simulink model "ground_state_nonridgid"  (R2017b)
settings: Solver=VariableStepAuto  StartTime=0.0  StopTime=10  RelTol=1e-3
undefined symbols (not defined in the file or in its folder): refo
settings Model: Creator=benma  LastModifiedBy=benma

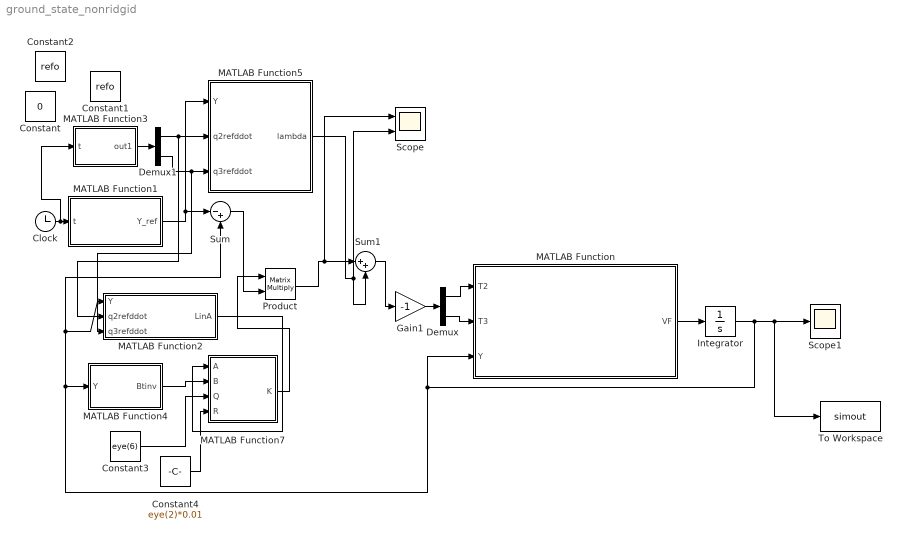
== system ground_state_nonridgid ==
  Clock : Clock
  Constant : Constant  Value=0
  Constant1 : Constant  Value=refo
  Constant2 : Constant  Value=refo
  Constant3 : Constant  Value=eye(6)
  Constant4 : Constant  Value=eye(2)*0.01
  Demux : Demux  Outputs=2
  Demux1 : Demux  Outputs=2
  Gain1 : Gain  Gain=-1
  Integrator : Integrator  InitialCondition=refo
  MATLAB Function : MATLAB Function  TreatAsAtomicUnit=on
  MATLAB Function1 : MATLAB Function  TreatAsAtomicUnit=on
  MATLAB Function2 : MATLAB Function  TreatAsAtomicUnit=on
  MATLAB Function3 : MATLAB Function  TreatAsAtomicUnit=on
  MATLAB Function4 : MATLAB Function  TreatAsAtomicUnit=on
  MATLAB Function5 : MATLAB Function  TreatAsAtomicUnit=on
  MATLAB Function7 : MATLAB Function  TreatAsAtomicUnit=on
  Product : Product  Multiplication=Matrix(*)
  Scope : Scope  NumInputPorts=2
  Scope1 : Scope
  Sum : Sum  Inputs=|-+
  Sum1 : Sum  Inputs=|++
  To Workspace : ToWorkspace  VariableName=simout  SaveFormat=Timeseries  SampleTime=-1
  wires:
  MATLAB Function/1(VF) -> Integrator/1
  Gain1/1 -> Demux/1
  Demux/1 -> MATLAB Function/1(T2)
  Demux/2 -> MATLAB Function/2(T3)
  MATLAB Function5/1(lambda) -> Sum1/2, Scope/2
  Sum1/1 -> Gain1/1
  Clock/1 -> MATLAB Function3/1(t), MATLAB Function1/1(t)
  MATLAB Function1/1(Y_ref) -> Sum/1, MATLAB Function5/1(Y)
  Integrator/1 -> To Workspace/1, Scope1/1, MATLAB Function/3(Y), MATLAB Function4/1(Y), MATLAB Function2/1(Y), Sum/2
  MATLAB Function2/1(LinA) -> MATLAB Function7/1(A)
  MATLAB Function4/1(Btinv) -> MATLAB Function7/2(B)
  Constant3/1 -> MATLAB Function7/3(Q)
  Constant4/1 -> MATLAB Function7/4(R)
  Product/1 -> Sum1/1, Scope/1
  Sum/1 -> Product/2
  MATLAB Function7/1(K) -> Product/1
  Demux1/1 -> MATLAB Function2/2(q2refddot), MATLAB Function5/2(q2refddot)
  MATLAB Function3/1(out1) -> Demux1/1
  Demux1/2 -> MATLAB Function2/3(q3refddot), MATLAB Function5/3(q3refddot)

== matlab function ground_state_nonridgid/MATLAB Function ==
  data: T2 input; VF output; T3 input; Y input
function VF = threedof_ground(T2,T3,Y)
%THREEDOF_GROUND
%    VF = THREEDOF_GROUND(T2,T3,Y)

%    This function was generated by the Symbolic Math Toolbox version 8.0.
%    23-Nov-2018 17:29:58

t2 = Y(2);
t3 = t2.*2.0;
t4 = Y(3);
t5 = t4.*2.0;
t6 = Y(1);
t7 = Y(4);
t8 = t7.^2;
t9 = t2-t4;
t10 = sin(t9);
t11 = Y(5);
t12 = Y(6);
t13 = t2+t5;
t14 = sin(t13);
t15 = t11.^2;
t16 = cos(t5);
t17 = cos(t13);
t18 = t3+t5;
t19 = sin(t2);
t20 = t2+t4;
t21 = sin(t20);
t22 = t12.^2;
t23 = cos(t2);
t24 = cos(t3);
t25 = t24.*8.1e1;
t26 = t16.*4.5e1;
t27 = cos(t18);
t66 = t27.*9.0;
t28 = t25+t26-t66-1.69e2;
t29 = 1.0./t28;
t30 = cos(t6);
t31 = t3+t6;
t32 = cos(t31);
t33 = t32.*1.32435e4;
t34 = -t5+t6;
t35 = cos(t34);
t36 = t35.*4.4145e3;
t37 = t5+t6;
t38 = cos(t37);
t39 = t38.*4.4145e3;
t40 = t3+t5+t6;
t41 = cos(t40);
t42 = sin(t3);
t43 = sin(t5);
t44 = t8.*t10.*4.5e2;
t45 = t10.*t15.*4.5e2;
t46 = t10.*t22.*4.5e2;
t47 = t3+t4;
t48 = sin(t47);
t49 = cos(t9);
t50 = T3.*t17.*9.0e2;
t51 = sin(t18);
t52 = t15.*t19.*2.25e3;
t53 = sin(t4);
t54 = t8.*t21.*2.5e2;
t55 = t15.*t21.*2.5e2;
t56 = t21.*t22.*2.5e2;
t57 = cos(t20);
t58 = T3.*t57.*2.1e3;
t59 = t7.*t11.*t21.*5.0e2;
t60 = t7.*t12.*t21.*5.0e2;
t61 = t11.*t12.*t21.*5.0e2;
t62 = t7.*t10.*t11.*9.0e2;
t63 = t7.*t10.*t12.*9.0e2;
t64 = t10.*t11.*t12.*9.0e2;
t65 = t7.*t11.*t19.*4.5e3;
t67 = t2+t6;
t68 = cos(t67);
t69 = t68.*2.20725e4;
t70 = t2+t5+t6;
t71 = cos(t70);
t72 = -t2+t6;
t73 = cos(t72);
t74 = t2+t5-t6;
t75 = cos(t74);
t76 = t75.*4.4145e3;
t77 = t8.*t42.*1.35e3;
t78 = t15.*t42.*1.35e3;
t79 = t22.*t48.*4.5e2;
t80 = cos(t47);
t81 = T3.*t27.*9.0e2;
t82 = T2.*t23.*2.7e3;
t83 = cos(t4);
t84 = t7.*t11.*t42.*2.7e3;
t85 = t7.*t12.*t48.*9.0e2;
t86 = t11.*t12.*t48.*9.0e2;
VF = [t7;t11;t12;t29.*(T2.*2.3e3-t30.*3.1392e4+t33+t36+t39-t41.*1.4715e3+t44+t45+t46+t50+t52+t54+t55+t56+t58+t59+t60+t61+t62+t63+t64+t65+t77+t82-T2.*t16.*9.0e2-T2.*t17.*9.0e2-T3.*t23.*2.7e3-T3.*t49.*2.7e3-t8.*t14.*1.5e2+t8.*t19.*2.25e3-t14.*t15.*1.5e2-t8.*t51.*1.5e2-t7.*t11.*t14.*3.0e2).*(-3.0./5.0e1);t29.*(T2.*7.0e3-T3.*4.7e3-t30.*3.1392e4+t33+t36+t39-t41.*1.4715e3+t44+t45+t46+t50+t52+t54+t55+t56+t58+t59+t60+t61+t62+t63+t64+t65+t69-t71.*2.943e3-t73.*2.6487e4+t76+t78+t79+t81+t84+t85+t86-T2.*t16.*9.0e2-T2.*t17.*1.8e3+T2.*t23.*5.4e3-T3.*t23.*2.7e3-T2.*t27.*9.0e2-T3.*t49.*2.7e3+T3.*t80.*2.7e3-T3.*t83.*5.7e3-t8.*t14.*9.0e2+t8.*t19.*7.2e3-t14.*t15.*1.5e2+t8.*t42.*2.7e3-t8.*t43.*7.5e2+t8.*t48.*4.5e2-t15.*t43.*7.5e2-t8.*t51.*1.5e2-t8.*t53.*1.45e3+t15.*t48.*4.5e2-t15.*t53.*1.45e3-t22.*t53.*1.45e3-t7.*t11.*t14.*3.0e2-t7.*t11.*t43.*1.5e3+t7.*t11.*t48.*9.0e2-t7.*t11.*t53.*2.9e3-t7.*t12.*t53.*2.9e3-t11.*t12.*t53.*2.9e3).*(3.0./5.0e1);t29.*(T2.*4.7e3-T3.*1.9e4+t69-t71.*2.943e3-t73.*2.6487e4+t76+t77+t78+t79+t81+t82+t84+t85+t86-cos(t2+t4+t6).*2.4525e3+cos(t2+t4-t6).*5.886e3+cos(t2-t4+t6).*8.829e3-cos(-t2+t4+t6).*1.32435e4-T2.*t17.*9.0e2+T3.*t24.*8.1e3-T2.*t27.*9.0e2+T2.*t49.*2.7e3-T2.*t57.*2.1e3-T2.*t80.*2.7e3+T3.*t80.*5.4e3+T2.*t83.*5.7e3-T3.*t83.*1.14e4+t8.*t10.*2.25e3-t8.*t14.*7.5e2+t8.*t19.*4.95e3-t8.*t21.*8.5e2-t8.*t43.*1.5e3+t8.*t48.*9.0e2-t15.*t43.*1.5e3+t8.*t51.*1.5e2-t8.*t53.*5.0e3+t15.*t48.*9.0e2-t22.*t43.*7.5e2+t15.*t51.*1.5e2-t15.*t53.*5.0e3+t22.*t51.*1.5e2-t22.*t53.*1.45e3-t7.*t11.*t43.*3.0e3-t7.*t12.*t43.*1.5e3+t7.*t11.*t48.*1.8e3-t11.*t12.*t43.*1.5e3+t7.*t11.*t51.*3.0e2+t7.*t12.*t51.*3.0e2-t7.*t11.*t53.*1.0e4-t7.*t12.*t53.*2.9e3+t11.*t12.*t51.*3.0e2-t11.*t12.*t53.*2.9e3).*(-3.0./5.0e1)];

== matlab function ground_state_nonridgid/MATLAB Function1 ==
  data: t input; Y_ref output
function Y_ref = Reference(t)
%REFERENCE
%    Y_REF = REFERENCE(T)

%    This function was generated by the Symbolic Math Toolbox version 8.0.
%    14-Jan-2019 20:45:13

t2 = t.*1.0e1;
t3 = exp(t2);
t4 = exp(-2.5e1);
t5 = t.^2;
t6 = exp(-t5);
t7 = t3.*t4.*t6.*pi.*(1.0./2.0);
t8 = cos(t7);
t9 = sin(t7);
t10 = t-5.0;
t11 = t10.^2;
t12 = exp(-t11);
t13 = t12.*pi.*(1.0./2.0);
t14 = t8+2.0;
t15 = t8.*4.0;
t16 = t8.^2;
t17 = t9.^2;
t18 = t15+t16+t17+4.0;
t19 = sqrt(t18);
t20 = t9-t19;
t21 = 1.0./t14;
t22 = t3.*t4.*t6.*pi.*5.0;
t24 = t.*t3.*t4.*t6.*pi;
t23 = t22-t24;
t25 = 1.0./t14.^2;
t26 = t.*2.0;
t27 = t26-1.0e1;
Y_ref = [atan(t20.*t21).*-2.0;t13;-t13;(t21.*(t8.*t23+t9.*1.0./sqrt(t18).*t23.*2.0).*-2.0-t9.*t20.*t23.*t25.*2.0)./(t20.^2.*t25+1.0);t12.*t27.*pi.*(-1.0./2.0);t12.*t27.*pi.*(1.0./2.0)];

== matlab function ground_state_nonridgid/MATLAB Function2 ==
  data: Y input; LinA output; q2refddot input; q3refddot input
function LinA = LinA(Y,q2refddot,q3refddot)
%LINA
%    LINA = LINA(Y,Q2REFDDOT,Q3REFDDOT)

%    This function was generated by the Symbolic Math Toolbox version 8.0.
%    14-Jan-2019 20:08:35

t2 = Y(2);
t3 = t2.*2.0;
t4 = Y(3);
t5 = t4.*2.0;
t6 = Y(1);
t7 = cos(t3);
t8 = t7.*8.1e1;
t9 = cos(t5);
t10 = t9.*4.5e1;
t11 = t3+t5;
t12 = cos(t11);
t172 = t12.*9.0;
t13 = t8+t10-t172-1.69e2;
t14 = 1.0./t13;
t15 = t3+t6;
t16 = sin(t15);
t17 = t3+t5+t6;
t18 = sin(t17);
t19 = Y(4);
t20 = t2-t4;
t21 = cos(t20);
t22 = Y(5);
t23 = t19.^2;
t24 = Y(6);
t25 = t2+t5;
t26 = cos(t25);
t27 = t22.^2;
t28 = cos(t2);
t29 = t2+t4;
t30 = cos(t29);
t31 = t24.^2;
t32 = sin(t3);
t33 = sin(t20);
t34 = sin(t25);
t35 = t3+t4;
t36 = sin(t35);
t37 = cos(t35);
t38 = sin(t11);
t39 = sin(t2);
t40 = sin(t29);
t41 = cos(t4);
t42 = sin(t4);
t43 = t28.*3.0;
t44 = t30+t41+t43+4.0;
t45 = 1.0./t44;
t46 = cos(t6);
t47 = t2+t6;
t48 = cos(t47);
t49 = t4+t6;
t50 = cos(t49);
t51 = t2+t4-t6;
t52 = cos(t51);
t53 = t3+t4+t6;
t54 = cos(t53);
t55 = -t4+t6;
t56 = cos(t55);
t57 = cos(t17);
t58 = t57.*4.4145e3;
t59 = t2+t4+t6;
t60 = cos(t59);
t61 = sin(t5);
t62 = t23.*t33.*2.7e3;
t63 = t23.*t38.*9.0e2;
t64 = t27.*t38.*4.5e2;
t65 = t31.*t38.*4.5e2;
t66 = t23.*t40.*9.9e3;
t67 = t19.*t22.*t38.*9.0e2;
t68 = t19.*t24.*t38.*9.0e2;
t69 = t22.*t24.*t38.*9.0e2;
t70 = q2refddot.*2.35e3;
t71 = q3refddot.*3.5e3;
t72 = t50.*4.4145e3;
t73 = t2-t4+t6;
t74 = cos(t73);
t75 = t54.*1.32435e4;
t76 = t2+t5+t6;
t77 = cos(t76);
t78 = t77.*4.4145e3;
t79 = t60.*2.943e4;
t80 = t23.*t61.*9.0e2;
t81 = t27.*t61.*9.0e2;
t82 = t31.*t61.*4.5e2;
t83 = t23.*t36.*2.7e3;
t84 = t23.*t34.*1.8e3;
t85 = t27.*t36.*1.35e3;
t86 = t27.*t34.*1.35e3;
t87 = t31.*t34.*9.0e2;
t88 = q2refddot.*t21.*1.35e3;
t89 = t27.*t39.*1.35e3;
t90 = t23.*t42.*9.9e3;
t91 = t27.*t42.*5.85e3;
t92 = t31.*t42.*6.0e2;
t93 = t27.*t40.*4.65e3;
t94 = t31.*t40.*6.0e2;
t95 = q2refddot.*t28.*1.35e3;
t96 = q2refddot.*t41.*2.85e3;
t97 = q3refddot.*t28.*2.7e3;
t98 = t19.*t22.*t40.*9.3e3;
t99 = t19.*t24.*t40.*1.2e3;
t100 = t22.*t24.*t40.*1.2e3;
t101 = t19.*t22.*t61.*1.8e3;
t102 = t19.*t24.*t61.*9.0e2;
t103 = t22.*t24.*t61.*9.0e2;
t104 = t19.*t22.*t36.*2.7e3;
t105 = t19.*t22.*t34.*2.7e3;
t106 = t19.*t24.*t34.*1.8e3;
t107 = t22.*t24.*t34.*1.8e3;
t108 = t19.*t22.*t39.*2.7e3;
t109 = t19.*t22.*t42.*1.17e4;
t110 = t19.*t24.*t42.*1.2e3;
t111 = t22.*t24.*t42.*1.2e3;
t116 = t52.*2.20725e4;
t139 = q2refddot.*t12.*4.5e2;
t140 = q3refddot.*t12.*4.5e2;
t160 = t46.*2.50155e4;
t161 = t48.*1.32435e4;
t162 = t74.*1.32435e4;
t163 = t56.*3.5316e4;
t164 = q2refddot.*t30.*1.05e3;
t165 = t27.*t33.*1.35e3;
t166 = q3refddot.*t9.*4.5e2;
t167 = q2refddot.*t37.*1.35e3;
t168 = q2refddot.*t26.*4.5e2;
t169 = q3refddot.*t26.*9.0e2;
t170 = t19.*t22.*t33.*2.7e3;
t112 = t58-t62+t63+t64+t65+t66+t67+t68+t69+t70+t71+t72+t75+t78+t79+t80+t81+t82+t83+t84+t85+t86+t87+t88+t89+t90+t91+t92+t93+t94+t95+t96+t97+t98+t99+t100+t101+t102+t103+t104+t105+t106+t107+t108+t109+t110+t111-t116-t139-t140-t160-t161-t162-t163-t164-t165-t166-t167-t168-t169-t170;
t113 = q2refddot.*9.5e3;
t114 = q3refddot.*2.35e3;
t115 = t48.*5.73885e4;
t117 = t54.*2.6487e4;
t118 = -t2+t6;
t119 = cos(t118);
t120 = cos(t15);
t121 = t120.*3.97305e4;
t122 = t60.*1.91295e4;
t123 = t23.*t32.*8.1e3;
t124 = t27.*t32.*4.05e3;
t125 = t27.*t33.*2.7e3;
t126 = t23.*t36.*5.4e3;
t127 = t23.*t34.*9.0e2;
t128 = t31.*t33.*1.35e3;
t129 = t27.*t36.*2.7e3;
t130 = t27.*t34.*9.0e2;
t131 = t31.*t36.*1.35e3;
t132 = t31.*t34.*4.5e2;
t133 = q3refddot.*t21.*1.35e3;
t134 = t23.*t39.*2.25e4;
t135 = t27.*t39.*9.9e3;
t136 = t31.*t39.*1.35e3;
t137 = t27.*t40.*5.7e3;
t138 = t31.*t40.*1.65e3;
t141 = q2refddot.*t41.*5.7e3;
t142 = q3refddot.*t28.*1.35e3;
t143 = q3refddot.*t41.*2.85e3;
t144 = t19.*t22.*t40.*1.14e4;
t145 = t19.*t24.*t40.*3.3e3;
t146 = t22.*t24.*t40.*3.3e3;
t147 = t19.*t22.*t32.*8.1e3;
t148 = t19.*t22.*t33.*5.4e3;
t149 = t19.*t24.*t33.*2.7e3;
t150 = t19.*t22.*t36.*5.4e3;
t151 = t19.*t22.*t34.*1.8e3;
t152 = t22.*t24.*t33.*2.7e3;
t153 = t19.*t24.*t36.*2.7e3;
t154 = t19.*t24.*t34.*9.0e2;
t155 = t22.*t24.*t36.*2.7e3;
t156 = t22.*t24.*t34.*9.0e2;
t157 = t19.*t22.*t39.*1.98e4;
t158 = t19.*t24.*t39.*2.7e3;
t159 = t22.*t24.*t39.*2.7e3;
t175 = t46.*1.03005e5;
t176 = t50.*3.09015e4;
t177 = t119.*6.62175e4;
t178 = t56.*3.09015e4;
t179 = q3refddot.*t30.*1.05e3;
t180 = q2refddot.*t7.*4.05e3;
t181 = q2refddot.*t37.*2.7e3;
t182 = q3refddot.*t37.*1.35e3;
t183 = q3refddot.*t26.*4.5e2;
t184 = t31.*t42.*2.85e3;
t185 = t19.*t24.*t42.*5.7e3;
t186 = t22.*t24.*t42.*5.7e3;
t171 = t58+t62+t63+t64+t65+t66+t67+t68+t69+t113+t114+t115-t116+t117+t121+t122+t123+t124+t125+t126+t127+t128+t129+t130+t131+t132+t133+t134+t135+t136+t137+t138-t139-t140+t141+t142+t143+t144+t145+t146+t147+t148+t149+t150+t151+t152+t153+t154+t155+t156+t157+t158+t159-t175-t176-t177-t178-t179-t180-t181-t182-t183-t184-t185-t186;
t173 = -t5+t6;
t174 = t5+t6;
t187 = sin(t173);
t188 = sin(t174);
t189 = t18.*2.943e3;
t190 = t21.*t23.*4.5e2;
t191 = t21.*t27.*4.5e2;
t192 = t21.*t31.*4.5e2;
t193 = t23.*t30.*2.5e2;
t194 = t27.*t30.*2.5e2;
t195 = t30.*t31.*2.5e2;
t196 = t19.*t22.*t30.*5.0e2;
t197 = t19.*t24.*t30.*5.0e2;
t198 = t22.*t24.*t30.*5.0e2;
t199 = t19.*t21.*t22.*9.0e2;
t200 = t19.*t21.*t24.*9.0e2;
t201 = t21.*t22.*t24.*9.0e2;
t202 = t40.*t45.*t112.*(7.0./1.2e1);
t203 = 1.0./t13.^2;
t204 = t120.*1.32435e4;
t205 = cos(t173);
t206 = t205.*4.4145e3;
t207 = cos(t174);
t208 = t207.*4.4145e3;
t209 = t23.*t32.*1.35e3;
t210 = t23.*t33.*4.5e2;
t211 = t27.*t33.*4.5e2;
t212 = t31.*t33.*4.5e2;
t213 = t23.*t39.*2.25e3;
t214 = t27.*t39.*2.25e3;
t215 = t23.*t40.*2.5e2;
t216 = t27.*t40.*2.5e2;
t217 = t31.*t40.*2.5e2;
t218 = t19.*t22.*t40.*5.0e2;
t219 = t19.*t24.*t40.*5.0e2;
t220 = t22.*t24.*t40.*5.0e2;
t221 = t21.*t45.*t112.*(3.0./4.0);
t222 = t19.*t22.*t33.*9.0e2;
t223 = t19.*t24.*t33.*9.0e2;
t224 = t22.*t24.*t33.*9.0e2;
t225 = t28.*t45.*t112.*(3.0./4.0);
t226 = t9.*t45.*t171.*(1.0./4.0);
t227 = t26.*t45.*t171.*(1.0./4.0);
t228 = t19.*t22.*t39.*4.5e3;
t257 = t46.*3.1392e4;
t258 = t57.*1.4715e3;
t259 = t27.*t34.*1.5e2;
t260 = t23.*t38.*1.5e2;
t261 = t26.*t45.*t112.*(1.0./4.0);
t262 = t19.*t22.*t34.*3.0e2;
t263 = t30.*t45.*t112.*(7.0./1.2e1);
t314 = t28.*t45.*t171.*(3.0./4.0);
t229 = t204+t206+t208+t209+t210+t211+t212+t213+t214+t215+t216+t217+t218+t219+t220+t221+t222+t223+t224+t225+t226+t227+t228-t257-t258-t259-t260-t261-t262-t263-t314-t23.*t34.*1.5e2-t45.*t171.*(2.3e1./3.6e1);
t230 = t19.*t39.*4.5e3;
t231 = t22.*t39.*4.5e3;
t232 = t19.*t40.*5.0e2;
t233 = t22.*t40.*5.0e2;
t234 = t24.*t40.*5.0e2;
t235 = t19.*t33.*9.0e2;
t236 = t22.*t33.*9.0e2;
t237 = t24.*t33.*9.0e2;
t238 = sin(t6);
t239 = t16.*1.32435e4;
t240 = t187.*4.4145e3;
t241 = t188.*4.4145e3;
t242 = sin(t47);
t243 = sin(t76);
t244 = t243.*2.943e3;
t245 = sin(t118);
t246 = t245.*2.6487e4;
t247 = t2+t5-t6;
t248 = sin(t247);
t249 = t248.*4.4145e3;
t250 = t12.*t23.*3.0e2;
t251 = t27.*t28.*2.25e3;
t252 = t34.*t45.*t171.*(1.0./2.0);
t253 = t34.*t45.*t112.*(1.0./4.0);
t254 = t19.*t22.*t28.*4.5e3;
t255 = t38.*1.8e1;
t256 = t32.*1.62e2;
t264 = t188.*8.829e3;
t265 = t26.*t27.*3.0e2;
t266 = t19.*t22.*t26.*6.0e2;
t267 = t38.*t45.*t112.*(1.0./2.0);
t268 = t45.*t61.*t171.*(1.0./2.0);
t269 = t61.*9.0e1;
t270 = t255-t269;
t271 = t48.*2.20725e4;
t272 = cos(t247);
t273 = t272.*4.4145e3;
t274 = t23.*t32.*2.7e3;
t275 = t27.*t32.*1.35e3;
t276 = t23.*t36.*4.5e2;
t277 = t27.*t36.*4.5e2;
t278 = t31.*t36.*4.5e2;
t279 = t45.*t112.*(4.7e1./3.6e1);
t280 = t23.*t39.*7.2e3;
t281 = t12.*t45.*t171.*(1.0./4.0);
t282 = t19.*t22.*t32.*2.7e3;
t283 = t19.*t22.*t36.*9.0e2;
t284 = t19.*t24.*t36.*9.0e2;
t285 = t22.*t24.*t36.*9.0e2;
t286 = t41.*t45.*t112.*(1.9e1./1.2e1);
t287 = t26.*t45.*t171.*(1.0./2.0);
t311 = t77.*2.943e3;
t312 = t119.*2.6487e4;
t313 = t31.*t42.*1.45e3;
t315 = t12.*t45.*t112.*(1.0./4.0);
t316 = t19.*t24.*t42.*2.9e3;
t317 = t22.*t24.*t42.*2.9e3;
t288 = -t127+t204+t206+t208+t210+t211+t212+t214+t215+t216+t217+t218+t219+t220+t221+t222+t223+t224+t225+t226+t228-t257-t258-t259-t260-t261-t262-t263+t271+t273+t274+t275+t276+t277+t278+t279+t280+t281+t282+t283+t284+t285+t286+t287-t311-t312-t313-t315-t316-t317-t23.*t42.*1.45e3-t27.*t42.*1.45e3-t23.*t61.*7.5e2-t27.*t61.*7.5e2-t45.*t171.*(3.5e1./1.8e1)-t19.*t22.*t42.*2.9e3-t19.*t22.*t61.*1.5e3-t37.*t45.*t112.*(3.0./4.0)-t28.*t45.*t171.*(3.0./2.0);
t289 = t19.*t32.*2.7e3;
t290 = t22.*t32.*2.7e3;
t291 = t19.*t36.*9.0e2;
t292 = t22.*t36.*9.0e2;
t293 = t24.*t36.*9.0e2;
t294 = sin(t51);
t295 = t294.*5.886e3;
t296 = -t2+t4+t6;
t297 = sin(t296);
t298 = t297.*1.32435e4;
t299 = sin(t73);
t300 = sin(t59);
t301 = t300.*2.4525e3;
t302 = t31.*t37.*9.0e2;
t303 = t7.*t23.*2.7e3;
t304 = t7.*t27.*2.7e3;
t305 = t7.*t19.*t22.*5.4e3;
t306 = t38.*t45.*t171.*(1.0./2.0);
t307 = t19.*t24.*t37.*1.8e3;
t308 = t22.*t24.*t37.*1.8e3;
t309 = t39.*t45.*t171.*(3.0./4.0);
t310 = t255-t256;
t318 = t248.*8.829e3;
t319 = t21.*t23.*2.25e3;
t320 = t23.*t37.*9.0e2;
t321 = t27.*t37.*9.0e2;
t322 = t12.*t27.*3.0e2;
t323 = t12.*t31.*3.0e2;
t324 = t31.*t41.*1.45e3;
t325 = t33.*t45.*t171.*(3.0./4.0);
t326 = t36.*t45.*t112.*(3.0./2.0);
t327 = t19.*t22.*t37.*1.8e3;
t328 = t12.*t19.*t22.*6.0e2;
t329 = t12.*t19.*t24.*6.0e2;
t330 = t12.*t22.*t24.*6.0e2;
t331 = t19.*t24.*t41.*2.9e3;
t332 = t22.*t24.*t41.*2.9e3;
t333 = t52.*5.886e3;
t334 = cos(t296);
t335 = t74.*8.829e3;
t336 = t23.*t33.*2.25e3;
t337 = t23.*t36.*9.0e2;
t338 = t27.*t36.*9.0e2;
t339 = t27.*t38.*1.5e2;
t340 = t31.*t38.*1.5e2;
t341 = t45.*t112.*(9.5e1./1.8e1);
t342 = t23.*t39.*4.95e3;
t343 = t19.*t22.*t36.*1.8e3;
t344 = t30.*t45.*t171.*(7.0./1.2e1);
t345 = t41.*t45.*t112.*(1.9e1./6.0);
t346 = t19.*t22.*t38.*3.0e2;
t347 = t19.*t24.*t38.*3.0e2;
t348 = t22.*t24.*t38.*3.0e2;
t349 = t37.*t45.*t171.*(3.0./4.0);
t350 = t60.*(-2.4525e3)+t209+t227+t260+t271+t273+t275+t278+t281+t282+t284+t285-t311-t312-t313-t314-t315-t316-t317+t333-t334.*1.32435e4+t335+t336+t337+t338+t339+t340+t341+t342+t343+t344+t345+t346+t347+t348+t349-t23.*t34.*7.5e2-t23.*t40.*8.5e2-t23.*t42.*5.0e3-t27.*t42.*5.0e3-t23.*t61.*1.5e3-t27.*t61.*1.5e3-t31.*t61.*7.5e2-t45.*t171.*(4.7e1./3.6e1)-t19.*t22.*t42.*1.0e4-t19.*t22.*t61.*3.0e3-t19.*t24.*t61.*1.5e3-t22.*t24.*t61.*1.5e3-t7.*t45.*t112.*(9.0./4.0)-t37.*t45.*t112.*(3.0./2.0)-t21.*t45.*t171.*(3.0./4.0)-t41.*t45.*t171.*(1.9e1./1.2e1);
t351 = t19.*t38.*3.0e2;
t352 = t22.*t38.*3.0e2;
t353 = t24.*t38.*3.0e2;
t354 = t19.*t36.*1.8e3;
t355 = t22.*t36.*1.8e3;
LinA = reshape([0.0,0.0,0.0,t14.*(t18.*(-1.4715e3)-t238.*3.1392e4+t239+t240+t241).*(3.0./5.0e1),t14.*(t18.*1.4715e3+t238.*3.1392e4-t239-t240-t241-t242.*2.20725e4+t244+t246+t249).*(3.0./5.0e1),t14.*(t242.*(-2.20725e4)+t244+t246+t249+t295+t298-t299.*8.829e3+t301).*(-3.0./5.0e1),0.0,0.0,0.0,t14.*(t16.*-2.6487e4+t189+t190+t191+t192+t193+t194+t195+t196+t197+t198+t199+t200+t201+t202+t251+t253+t254+t303+t309-t12.*t23.*3.0e2-t23.*t26.*1.5e2+t23.*t28.*2.25e3-t26.*t27.*1.5e2-t19.*t22.*t26.*3.0e2-t33.*t45.*t112.*(3.0./4.0)-t39.*t45.*t112.*(3.0./4.0)-t34.*t45.*t171.*(1.0./4.0)).*(-3.0./5.0e1)+t203.*t229.*(t38.*1.8e1-t256).*(3.0./5.0e1),t14.*(t16.*-2.6487e4+t189+t190+t191+t192+t193+t194+t195+t196+t197+t198+t199+t200+t201+t202-t242.*2.20725e4+t244-t246-t249-t250+t251-t252+t253+t254+t267+t302+t304+t305+t307+t308+t320+t321+t326+t327+t7.*t23.*5.4e3-t23.*t26.*9.0e2+t23.*t28.*7.2e3-t26.*t27.*1.5e2-t19.*t22.*t26.*3.0e2-t33.*t45.*t112.*(3.0./4.0)-t39.*t45.*t112.*(3.0./4.0)-t38.*t45.*t171.*(1.0./2.0)+t39.*t45.*t171.*(3.0./2.0)).*(3.0./5.0e1)-t203.*t288.*t310.*(3.0./5.0e1),t14.*(t242.*(-2.20725e4)+t244-t246-t249+t250+t267-t295-t298-t299.*8.829e3+t301+t302+t303+t304+t305-t306+t307+t308+t309+t319+t322+t323+t325+t328+t329+t330-t23.*t26.*7.5e2+t23.*t28.*4.95e3-t23.*t30.*8.5e2+t23.*t37.*1.8e3+t27.*t37.*1.8e3+t19.*t22.*t37.*3.6e3+t32.*t45.*t112.*(9.0./2.0)+t36.*t45.*t112.*3.0-t34.*t45.*t171.*(1.0./4.0)-t36.*t45.*t171.*(3.0./2.0)-t40.*t45.*t171.*(7.0./1.2e1)).*(-3.0./5.0e1)+t203.*t310.*t350.*(3.0./5.0e1),0.0,0.0,0.0,t14.*(t187.*-8.829e3-t189+t190+t191+t192-t193-t194-t195-t196-t197-t198+t199+t200+t201-t202+t250+t252+t264+t265+t266+t268+t23.*t26.*3.0e2-t33.*t45.*t112.*(3.0./4.0)-t34.*t45.*t112.*(1.0./2.0)).*(3.0./5.0e1)+t203.*t229.*t270.*(3.0./5.0e1),t14.*(t187.*-8.829e3-t189+t190+t191+t192-t193-t194-t195-t196-t197-t198+t199+t200+t201-t202-t243.*5.886e3+t250+t264+t265+t266-t267+t268+t306+t318+t324+t331+t332+t9.*t23.*1.5e3+t9.*t27.*1.5e3+t23.*t26.*1.8e3-t23.*t37.*4.5e2+t23.*t41.*1.45e3-t27.*t37.*4.5e2+t27.*t41.*1.45e3-t31.*t37.*4.5e2+t9.*t19.*t22.*3.0e3-t19.*t22.*t37.*9.0e2-t19.*t24.*t37.*9.0e2+t19.*t22.*t41.*2.9e3-t22.*t24.*t37.*9.0e2-t33.*t45.*t112.*(3.0./4.0)-t34.*t45.*t112.*(1.0./2.0)-t36.*t45.*t112.*(3.0./4.0)+t42.*t45.*t112.*(1.9e1./1.2e1)+t34.*t45.*t171).*(-3.0./5.0e1)-t203.*t270.*t288.*(3.0./5.0e1),t14.*(t243.*-5.886e3-t250+t252-t267+t295-t298-t299.*8.829e3-t301+t306+t318+t319-t320-t321-t322-t323+t324+t325-t326-t327-t328-t329-t330+t331+t332+t9.*t23.*3.0e3+t9.*t27.*3.0e3+t9.*t31.*1.5e3+t23.*t26.*1.5e3+t23.*t30.*8.5e2+t23.*t41.*5.0e3+t27.*t41.*5.0e3-t31.*t37.*4.5e2+t9.*t19.*t22.*6.0e3+t9.*t19.*t24.*3.0e3+t9.*t22.*t24.*3.0e3-t19.*t24.*t37.*9.0e2+t19.*t22.*t41.*1.0e4-t22.*t24.*t37.*9.0e2+t42.*t45.*t112.*(1.9e1./6.0)+t36.*t45.*t171.*(3.0./4.0)+t40.*t45.*t171.*(7.0./1.2e1)-t42.*t45.*t171.*(1.9e1./1.2e1)).*(3.0./5.0e1)+t203.*t270.*t350.*(3.0./5.0e1),1.0,0.0,0.0,t14.*(t230+t231+t232+t233+t234+t235+t236+t237+t289-t19.*t34.*3.0e2-t22.*t34.*3.0e2-t19.*t38.*3.0e2).*(-3.0./5.0e1),t14.*(t231+t232+t233+t234+t235+t236+t237+t290+t291+t292+t293+t19.*t32.*5.4e3-t19.*t34.*1.8e3-t22.*t34.*3.0e2-t19.*t38.*3.0e2+t19.*t39.*1.44e4-t19.*t42.*2.9e3-t22.*t42.*2.9e3-t24.*t42.*2.9e3-t19.*t61.*1.5e3-t22.*t61.*1.5e3).*(3.0./5.0e1),t14.*(t289+t290+t293+t351+t352+t353+t354+t355+t19.*t33.*4.5e3-t19.*t34.*1.5e3+t19.*t39.*9.9e3-t19.*t40.*1.7e3-t19.*t42.*1.0e4-t22.*t42.*1.0e4-t24.*t42.*2.9e3-t19.*t61.*3.0e3-t22.*t61.*3.0e3-t24.*t61.*1.5e3).*(-3.0./5.0e1),0.0,1.0,0.0,t14.*(t230+t231+t232+t233+t234+t235+t236+t237-t19.*t34.*3.0e2-t22.*t34.*3.0e2).*(-3.0./5.0e1),t14.*(t230+t231+t232+t233+t234+t235+t236+t237+t289+t290+t291+t292+t293-t19.*t34.*3.0e2-t22.*t34.*3.0e2-t19.*t42.*2.9e3-t22.*t42.*2.9e3-t24.*t42.*2.9e3-t19.*t61.*1.5e3-t22.*t61.*1.5e3).*(3.0./5.0e1),t14.*(t289+t290+t293+t351+t352+t353+t354+t355-t19.*t42.*1.0e4-t22.*t42.*1.0e4-t24.*t42.*2.9e3-t19.*t61.*3.0e3-t22.*t61.*3.0e3-t24.*t61.*1.5e3).*(-3.0./5.0e1),0.0,0.0,1.0,t14.*(t232+t233+t234+t235+t236+t237).*(-3.0./5.0e1),t14.*(t232+t233+t234+t235+t236+t237+t291+t292+t293-t19.*t42.*2.9e3-t22.*t42.*2.9e3-t24.*t42.*2.9e3).*(3.0./5.0e1),t14.*(t291+t292+t293+t351+t352+t353-t19.*t42.*2.9e3-t22.*t42.*2.9e3-t24.*t42.*2.9e3-t19.*t61.*1.5e3-t22.*t61.*1.5e3-t24.*t61.*1.5e3).*(-3.0./5.0e1)],[6,6]);

== matlab function ground_state_nonridgid/MATLAB Function3 ==
  data: t input; out1 output
function out1 = refddot(t)
%REFDDOT
%    OUT1 = REFDDOT(T)

%    This function was generated by the Symbolic Math Toolbox version 8.0.
%    14-Jan-2019 20:51:15

t2 = t-5.0;
t3 = t2.^2;
t4 = exp(-t3);
t6 = t.*2.0;
t5 = t6-1.0e1;
t7 = t5.^2;
t8 = t4.*t7.*pi.*(1.0./2.0);
out1 = [t8-t4.*pi;-t8+t4.*pi];

== matlab function ground_state_nonridgid/MATLAB Function5 ==
  data: Y input; lambda output; q2refddot input; q3refddot input
function lambda = nonridgid_torque(Y,q2refddot,q3refddot)
%NONRIDGID_TORQUE
%    LAMBDA = NONRIDGID_TORQUE(Y,Q2REFDDOT,Q3REFDDOT)

%    This function was generated by the Symbolic Math Toolbox version 8.0.
%    14-Jan-2019 19:30:09

t2 = Y(2);
t3 = Y(3);
t4 = Y(1);
t5 = t2.*2.0;
t6 = Y(4);
t7 = sin(t5);
t8 = Y(5);
t9 = t2+t3;
t10 = cos(t9);
t11 = t6.^2;
t12 = t2-t3;
t13 = sin(t12);
t14 = t8.^2;
t15 = t3.*2.0;
t16 = Y(6);
t17 = t3+t5;
t18 = sin(t17);
t19 = t2+t15;
t20 = sin(t19);
t21 = t16.^2;
t22 = cos(t17);
t23 = t5+t15;
t24 = sin(t23);
t25 = sin(t2);
t26 = sin(t9);
t27 = cos(t23);
t28 = cos(t3);
t29 = cos(t2);
t30 = sin(t3);
t31 = t29.*3.0;
t32 = t10+t28+t31+4.0;
t33 = 1.0./t32;
t34 = cos(t4);
t35 = t2+t4;
t36 = cos(t35);
t37 = t3+t4;
t38 = cos(t37);
t39 = t2+t3-t4;
t40 = cos(t39);
t41 = t3+t4+t5;
t42 = cos(t41);
t43 = -t3+t4;
t44 = cos(t43);
t45 = t4+t5+t15;
t46 = cos(t45);
t47 = t46.*4.4145e3;
t48 = t2+t3+t4;
t49 = cos(t48);
t50 = sin(t15);
t51 = t11.*t13.*2.7e3;
t52 = cos(t12);
t53 = cos(t19);
t54 = t11.*t24.*9.0e2;
t55 = t14.*t24.*4.5e2;
t56 = t21.*t24.*4.5e2;
t57 = t11.*t26.*9.9e3;
t58 = t6.*t8.*t24.*9.0e2;
t59 = t6.*t16.*t24.*9.0e2;
t60 = t8.*t16.*t24.*9.0e2;
lambda = [t33.*(q2refddot.*9.5e3+q3refddot.*2.35e3-t34.*1.03005e5+t36.*5.73885e4-t38.*3.09015e4-t40.*2.20725e4+t42.*2.6487e4-t44.*3.09015e4+t47+t49.*1.91295e4+t51+t54+t55+t56+t57+t58+t59+t60-cos(-t2+t4).*6.62175e4+cos(t4+t5).*3.97305e4-q3refddot.*t10.*1.05e3-q2refddot.*t22.*2.7e3-q3refddot.*t22.*1.35e3-q2refddot.*t27.*4.5e2+q2refddot.*t28.*5.7e3-q3refddot.*t27.*4.5e2+q3refddot.*t28.*2.85e3+q3refddot.*t29.*1.35e3+q3refddot.*t52.*1.35e3-q3refddot.*t53.*4.5e2+t7.*t11.*8.1e3+t7.*t14.*4.05e3+t13.*t14.*2.7e3+t11.*t18.*5.4e3+t11.*t20.*9.0e2+t14.*t18.*2.7e3+t13.*t21.*1.35e3+t14.*t20.*9.0e2+t11.*t25.*2.25e4+t14.*t25.*9.9e3+t18.*t21.*1.35e3+t14.*t26.*5.7e3+t20.*t21.*4.5e2+t21.*t25.*1.35e3+t21.*t26.*1.65e3-t21.*t30.*2.85e3-q2refddot.*cos(t5).*4.05e3+t6.*t7.*t8.*8.1e3+t6.*t8.*t13.*5.4e3+t6.*t8.*t18.*5.4e3+t6.*t8.*t20.*1.8e3+t6.*t13.*t16.*2.7e3+t8.*t13.*t16.*2.7e3+t6.*t8.*t25.*1.98e4+t6.*t8.*t26.*1.14e4+t6.*t16.*t18.*2.7e3+t6.*t16.*t20.*9.0e2+t8.*t16.*t18.*2.7e3+t8.*t16.*t20.*9.0e2+t6.*t16.*t25.*2.7e3+t6.*t16.*t26.*3.3e3+t8.*t16.*t25.*2.7e3+t8.*t16.*t26.*3.3e3-t6.*t16.*t30.*5.7e3-t8.*t16.*t30.*5.7e3).*2.777777777777778e-4;t33.*(q2refddot.*2.35e3+q3refddot.*3.5e3-t34.*2.50155e4-t36.*1.32435e4+t38.*4.4145e3-t40.*2.20725e4+t42.*1.32435e4-t44.*3.5316e4+t47+t49.*2.943e4-t51+t54+t55+t56+t57+t58+t59+t60+cos(t2+t4+t15).*4.4145e3-cos(t2-t3+t4).*1.32435e4-q2refddot.*t10.*1.05e3-q2refddot.*t22.*1.35e3-q2refddot.*t27.*4.5e2+q2refddot.*t28.*2.85e3-q3refddot.*t27.*4.5e2+q2refddot.*t29.*1.35e3+q3refddot.*t29.*2.7e3+q2refddot.*t52.*1.35e3-q2refddot.*t53.*4.5e2-q3refddot.*t53.*9.0e2-t13.*t14.*1.35e3+t11.*t18.*2.7e3+t11.*t20.*1.8e3+t14.*t18.*1.35e3+t14.*t20.*1.35e3+t14.*t25.*1.35e3+t14.*t26.*4.65e3+t11.*t30.*9.9e3+t20.*t21.*9.0e2+t14.*t30.*5.85e3+t21.*t26.*6.0e2+t21.*t30.*6.0e2+t11.*t50.*9.0e2+t14.*t50.*9.0e2+t21.*t50.*4.5e2-q3refddot.*cos(t15).*4.5e2-t6.*t8.*t13.*2.7e3+t6.*t8.*t18.*2.7e3+t6.*t8.*t20.*2.7e3+t6.*t8.*t25.*2.7e3+t6.*t8.*t26.*9.3e3+t6.*t16.*t20.*1.8e3+t6.*t8.*t30.*1.17e4+t8.*t16.*t20.*1.8e3+t6.*t16.*t26.*1.2e3+t8.*t16.*t26.*1.2e3+t6.*t16.*t30.*1.2e3+t8.*t16.*t30.*1.2e3+t6.*t8.*t50.*1.8e3+t6.*t16.*t50.*9.0e2+t8.*t16.*t50.*9.0e2).*2.777777777777778e-4];

== matlab function ground_state_nonridgid/MATLAB Function4 ==
  data: Y input; Btinv output
function Btinv = LinB(Y)
%LINB
%    BTINV = LINB(Y)

%    This function was generated by the Symbolic Math Toolbox version 8.0.
%    15-Dec-2018 02:08:11

t2 = Y(2);
t3 = t2.*2.0;
t4 = Y(3);
t5 = t4.*2.0;
t6 = cos(t5);
t7 = cos(t2);
t8 = t2+t5;
t9 = cos(t8);
t10 = t9.*9.0e2;
t11 = cos(t3);
t12 = t11.*8.1e1;
t13 = t6.*4.5e1;
t14 = t3+t5;
t15 = cos(t14);
t18 = t15.*9.0;
t16 = t12+t13-t18-1.69e2;
t17 = 1.0./t16;
t19 = t6.*9.0e2;
t20 = t7.*2.7e3;
t21 = t2+t4;
t22 = cos(t21);
t23 = t22.*2.1e3;
t24 = t2-t4;
t25 = cos(t24);
t26 = t15.*9.0e2;
t27 = cos(t4);
t28 = t3+t4;
t29 = cos(t28);
t30 = t29.*2.7e3;
t31 = t17.*(t10-t20+t23-t25.*2.7e3+t26-t27.*5.7e3+t30-4.7e3).*(3.0./5.0e1);
Btinv = reshape([0.0,0.0,0.0,t17.*(t10+t19-t20-2.3e3).*(3.0./5.0e1),t17.*(t7.*-5.4e3+t9.*1.8e3+t19+t26-7.0e3).*(-3.0./5.0e1),t31,0.0,0.0,0.0,t17.*(t10-t20+t23-t25.*2.7e3).*(-3.0./5.0e1),t31,t17.*(t11.*8.1e3+t26-t27.*1.14e4+t29.*5.4e3-1.9e4).*(-3.0./5.0e1)],[6,2]);

== matlab function ground_state_nonridgid/MATLAB Function7 ==
  data: A input; K output; B input; Q input; R input
function K = SDLQR(A,B,Q,R)
coder.extrinsic('ordschur')
H=[double(A) -double(B)*inv(R)*double(B.');
    -Q -double(A.')];
[n,m]=size(A);
[z,t] = schur(H,'real');
[z,t,Success] = ordschur(z,t,'lhp');
X1 = z(1:n,1:n);
X2 = z(n+1:n*2,1:n);
X=X2*inv(X1);
dB = double(B);
K = inv(R)*dB.'*X;
K=K
